simulink model "SimulationModel"  (R2020a)
settings: Solver=VariableStepAuto  StartTime=0.0  StopTime=10.0  RelTol=1e-3
libraries: cstblocks x2
settings Model: Creator=Strel  LastModifiedBy=Strel

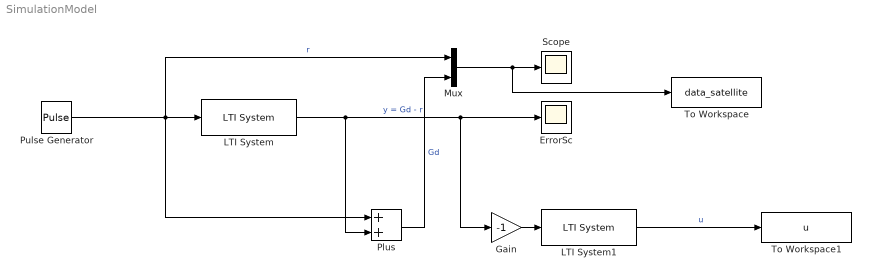
== system SimulationModel ==
  ErrorSc : Scope
  Gain : Gain  Gain=-1
  LTI System : cstblocks/LTI System  sys=ssys  IC=[]
  LTI System1 : cstblocks/LTI System  sys=Kd  IC=[]
  Mux : Mux  Inputs=2
  Plus : Sum
  Pulse Generator : DiscretePulseGenerator  PulseType=Time based  Period=10  PulseWidth=50
  Scope : Scope
  To Workspace : ToWorkspace  VariableName=data_satellite  SaveFormat=Timeseries  SampleTime=-1
  To Workspace1 : ToWorkspace  VariableName=u  SaveFormat=Timeseries  SampleTime=-1
  wires:
  LTI System1/1 -> To Workspace1/1  "u"
  Mux/1 -> To Workspace/1, Scope/1
  LTI System/1 -> Plus/2, Gain/1, ErrorSc/1  "y = Gd - r"
  Plus/1 -> Mux/2  "Gd"
  Pulse Generator/1 -> Mux/1, Plus/1, LTI System/1  "r"
  Gain/1 -> LTI System1/1
